simulink model "QD2_IMU_2021a"  (R2021a)
settings: Solver=ode2  StartTime=0.0  StopTime=inf  FixedStep=1/1000  RelTol=1e-3  EnableMultiTasking=on
undefined symbols (not defined in the file): HIL
libraries: quarc_library x7, simulink x2
settings Model: DataTypeOverride=Double  MinMaxOverflowLogging=ForceOff  SimulationMode=external  ExtModeTrigElement=1  ExtModeTrigDuration=10000  ExtModeTrigLevel=0.400000  Creator=dmadill  LastModifiedBy=lgonzalez
settings SolverCC: AlgebraicLoopSolver=TrustRegion  PositivePriorityOrder=on
settings DataIOCC: ReturnWorkspaceOutputs=off
settings DebuggingCC: SFMachineParentedDataDiag=warning  ArithmeticOperatorsInVariantConditions=warning
settings HardwareCC: ProdBitPerLong=64  ProdLargestAtomicInteger=LongLong  ProdLargestAtomicFloat=Double  ProdLongLongMode=on  ProdHWDeviceType=ARM Compatible->ARM 64-bit (LP64)
settings SFSimCC: SimUseLocalCustomCode=off  CustomCodeUndefinedFunction=UseInterfaceOnly
settings RTWCC: Description=QUARC Linux QDrone2 Target Using Toolchain  SystemTargetFile=quarc_linux_qdrone2.tlc  RTWUseLocalCustomCode=off  Toolchain=QUARC linux_qdrone2 | gmake (64-bit Windows)  BuildConfiguration=Faster Runs
settings CodeAppCC: StateflowObjectComments=on
settings STFCustomTargetCC: ConcurrentExecutionCompliant=on  SystemTargetFile=quarc_linux_qdrone2.tlc
settings GRTTargetCC: TargetLangStandard=C89/C90 (ANSI)  ParMdlRefBuildCompliant=off  CompOptLevelCompliant=off  CombineOutputUpdateFcns=off  MatFileLogging=off  CPPClassGenCompliant=off  GRTInterface=on  ExtMode=on  ExtModeMexFile=quarc_comm  ExtModeMexArgs='-w -d /tmp -uri %u','tcpip://192.168.2.d:17001'
settings ConfigComp: CovMetricSettings=dswe

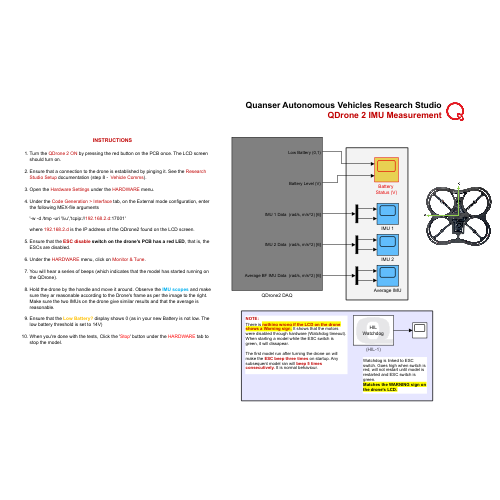
[thumbnail: Simulink's stored preview of the top-level diagram]
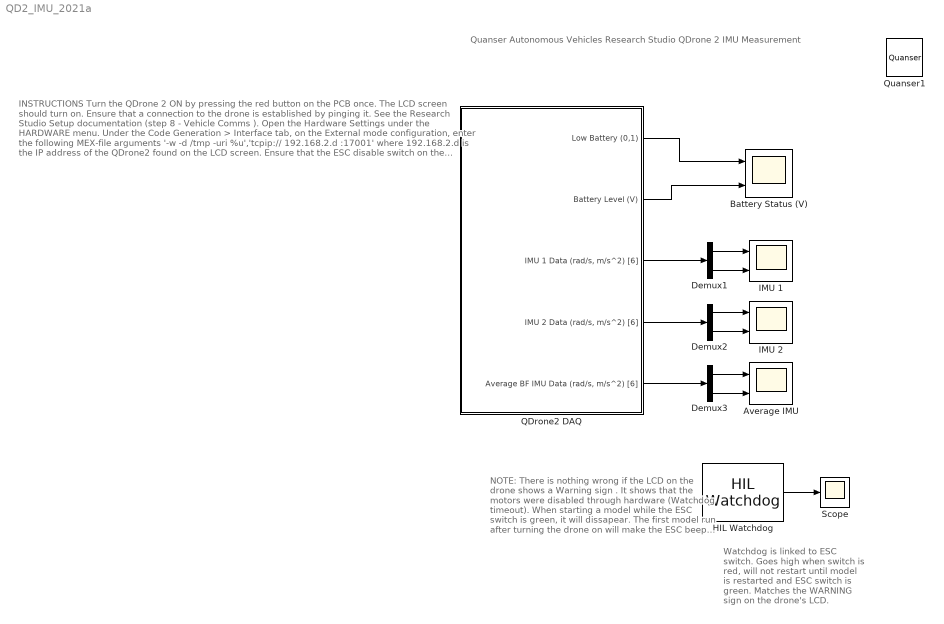
== system QD2_IMU_2021a ==
  note: Quanser Autonomous Vehicles Research Studio
      | QDrone 2 IMU Measurement
  note: Watchdog is linked to ESC switch. Goes high when switch is red, will not restart until model is restarted and ESC switch is green.
      | Matches the WARNING sign on the drone's LCD.
  note: NOTE:
      | There is nothing wrong if the LCD on the drone shows a Warning sign . It shows that the motors were disabled through hardware (Watchdog timeout). When starting a model while the ESC switch is green, it will dissapear.
      |
      | The first model run after turning the drone on will make the ESC beep three times on startup. Any subsequent model ran will beep 5 times consecutively. It is normal behaviour.
  note: INSTRUCTIONS
      |
      | Turn the QDrone 2 ON by pressing the red button on the PCB once. The LCD screen should turn on.
      |
      | Ensure that a connection to the drone is established by pinging it. See the Research Studio Setup documentation (step 8 - Vehicle Comms ).
      |
      | Open the Hardware Settings under the HARDWARE menu.
      |
      | Under the Code Generation > Interface tab, on the External mode configuration, enter the following MEX-file arguments
      |
      | '-w -d /tmp -uri %u','tcpip:// 192.168.2.d :17001'
      |
      | where 192.168.2.d is the IP address of the QDrone2 found on the LCD screen.
      |
      | Ensure that the ESC disable switch on the drone's PCB has a red LED , that is, the ESCs are disabled.
      |
      | Under the HARDWARE menu, click on Monitor & Tune .
      |
      | You will hear a series of beeps (which indicates that the model has started running on the QDrone).
      |
      | Hold the drone by the handle and move it around. Observe the IMU scopes and make sure they ar reasonable according to the Drone's frame as per the image to the right. Make sure the two IMUs on the drone give similar results and that the average is reasonable.
      |
      | Ensure that the Low Battery? display shows 0 (as in your new Battery is not low. The low battery threshold is set to 14V)
      |
      | When you're done with the tests, Click the ' Stop ' button under the HARDWARE tab to stop the model.
  Average IMU : Scope  NumInputPorts=2
  Battery Status (V) : Scope  NumInputPorts=2
  Demux1 : Demux  Outputs=2
  Demux2 : Demux  Outputs=2
  Demux3 : Demux  Outputs=2
  HIL Watchdog : quarc_library/Data Acquisition/Generic/Watchdog/HIL Watchdog  object_name=HIL-1  timeout=0.1  sample_time=qc_get_step_size  active=off
      settings: AttributesFormatString=(%<object_name>)  SourceProductName=QUARC Targets
  IMU 1 : Scope  NumInputPorts=2
  IMU 2 : Scope  NumInputPorts=2
  QDrone2 DAQ : Subsystem
  Quanser1 : quarc_library/Logos/Quanser
  Scope : Scope
  wires:
  QDrone2 DAQ/1(Low Battery (0,1)) -> Battery Status (V)/1
  QDrone2 DAQ/2(Battery Level (V)) -> Battery Status (V)/2
  HIL Watchdog/1 -> Scope/1
  QDrone2 DAQ/3("IMU 1 Data (rad/s, m/s^2) [6]") -> Demux1/1
  QDrone2 DAQ/4("IMU 2 Data (rad/s, m/s^2) [6]") -> Demux2/1
  Demux1/1 -> IMU 1/1
  Demux1/2 -> IMU 1/2
  Demux2/1 -> IMU 2/1
  Demux2/2 -> IMU 2/2
  Demux3/1 -> Average IMU/1
  Demux3/2 -> Average IMU/2
  QDrone2 DAQ/5("Average BF IMU Data (rad/s, m/s^2) [6]") -> Demux3/1

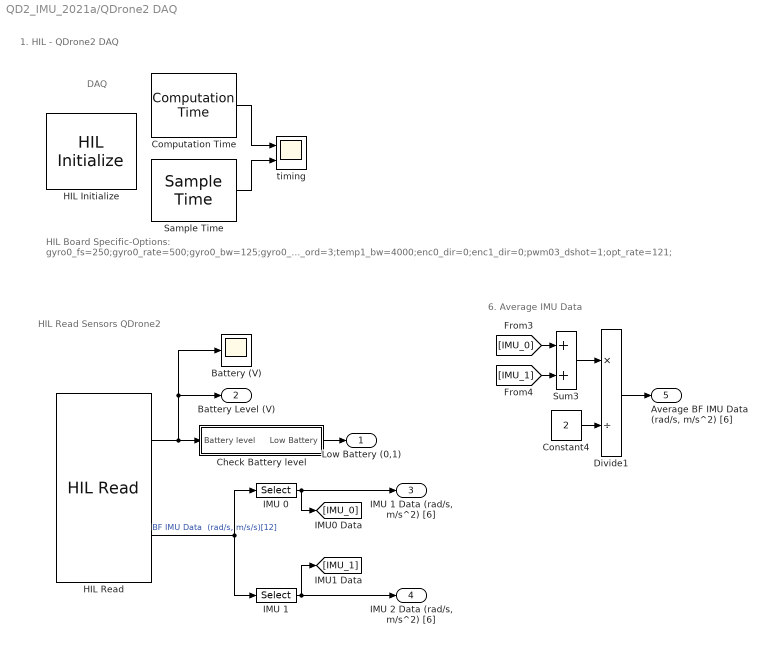
== system QD2_IMU_2021a/QDrone2 DAQ ==
  note: 1. HIL - QDrone2 DAQ
  note: DAQ
  note: HIL Read Sensors QDrone2
  note: 6. Average IMU Data
  note: HIL Board Specific-Options:
      | gyro0_fs=250;gyro0_rate=500;gyro0_bw=125;gyro0_ord=3;accel0_fs=16;accel0_rate=1000;accel0_bw=400;accel0_ord=3;temp0_bw=4000;gyro1_fs=250;gyro1_rate=500;gyro1_bw=125;gyro1_ord=3;accel1_fs=16;accel1_rate=1000;accel1_bw=400;accel1_ord=3;temp1_bw=4000;enc0_dir=0;enc1_dir=0;pwm03_dshot=1;opt_rate=121;
  Battery (V) : Scope
  Check Battery level : Subsystem
  Computation Time : quarc_library/Sources/Time/Computation Time  sample_time=qc_get_step_size  use_model=on  use_cpu_time=off
  Constant4 : Constant  Value=2
  Divide1 : Product  Inputs=*/
  HIL Initialize : quarc_library/Data Acquisition/Generic/Configuration/HIL Initialize  object_name=HIL-1  board_type=qdrone2  board_number=0  board_options=gyro0_fs=250;gyro0_rate=500;gyro0_bw=125;gyro0_ord=3;accel0_fs=16;accel0_rate=1000;accel0_bw=400;accel0_ord=3;temp0_bw=4000;gyro1_fs=250;gyro1_rate=500;gyro1_bw=125;gyro1_ord=3;accel1_fs=16;accel1_rate=1000;accel1_bw=400;accel1_ord=3;temp1_bw=4000;enc0_dir=0;enc1_dir=0;pwm03_dshot=1;opt_rate=121;  exclusive=off  active=on  hardware_clocks=[]  clock_modes=[]  initial_clock_frequencies=[]  set_clock_params_at_start=off  set_clock_params_at_switch_in=off  set_clock_frequencies_at_start=off  set_clock_frequencies_at_switch_in=off  analog_input_channels=[0:3]  analog_input_configurations=[]  analog_input_maximums=[3.3]  analog_input_minimums=[0]  set_analog_input_params_at_start=off  set_analog_input_params_at_switch_in=off  analog_output_channels=[]  analog_output_maximums=[]  analog_output_minimums=[]  initial_analog_outputs=[]  final_analog_outputs=[]  watchdog_analog_outputs=[]  set_analog_output_params_at_start=off  set_analog_output_params_at_switch_in=off  set_analog_outputs_at_start=off  set_analog_outputs_at_switch_in=off  set_analog_outputs_at_terminate=off  set_analog_outputs_at_switch_out=off  set_analog_outputs_on_watchdog=off  digital_input_channels=[0:5]  digital_output_channels=[6:11]  digital_output_configuration=[]  initial_digital_outputs=[0]  final_digital_outputs=[0]  watchdog_digital_outputs=[0 0 0 0 0 0]  set_digital_output_params_at_start=off  set_digital_output_params_at_switch_in=off  set_digital_outputs_at_start=on  set_digital_outputs_at_switch_in=off  set_digital_outputs_at_terminate=on  set_digital_outputs_at_switch_out=off  set_digital_outputs_on_watchdog=off  encoder_channels=[0:1]  quadrature=[4]  encoder_filter_frequency=100e6/1  initial_encoder_counts=[0]  set_encoder_params_at_start=on  set_encoder_params_at_switch_in=off  set_encoder_counts_at_start=on  set_encoder_counts_at_switch_in=off  pwm_channels=[0:5]  pwm_modes=[6 6 6 6 0 0]  pwm_frequency=1.2e6  pwm_configuration=[0]  pwm_alignment=[0]  pwm_polarity=[1]  pwm_leading_deadband=[]  pwm_trailing_deadband=[]  initial_pwm_outputs=[0]  final_pwm_outputs=[0]  watchdog_pwm_outputs=[0]  set_pwm_params_at_start=on  set_pwm_params_at_switch_in=off  set_pwm_outputs_at_start=on  set_pwm_outputs_at_switch_in=off  set_pwm_outputs_at_terminate=on  set_pwm_outputs_at_switch_out=off  set_pwm_outputs_on_watchdog=on  other_output_channels=[]  initial_other_outputs=[]  final_other_outputs=[]  watchdog_other_outputs=[]  set_other_outputs_at_start=on  set_other_outputs_at_switch_in=off  set_other_outputs_at_terminate=on  set_other_outputs_at_switch_out=off  set_other_outputs_on_watchdog=off
  HIL Read : quarc_library/Data Acquisition/Generic/Immediate I//O/HIL Read  object_name=HIL-1  analog_channels=[3]  encoder_channels=[]  digital_channels=[]  other_channels=[3000:3002 4000:4002 3003:3005 4003:4005]  sample_time=qc_get_step_size  active=on  vector_output=on  data_type_mode=Inherit via back propagation  encoder_data_type=double  digital_data_type=boolean
  IMU 0 : Selector  InputPortWidth=12  IndexOptions=Index vector (dialog)  Indices=[1:6]  OutputSizes=1
  IMU 1 : Selector  InputPortWidth=12  IndexOptions=Index vector (dialog)  Indices=[7:12]  OutputSizes=1
  Sample Time : quarc_library/Sources/Time/Sample Time  Priority=-99  sample_time=qc_get_step_size
  Sum3 : Sum
  timing : Scope  NumInputPorts=2
  Low Battery (0,1) : Outport
  Battery Level (V) : Outport  Port=2
  "IMU 1 Data (rad/s, m/s^2) [6]" : Outport  Port=3
  "IMU 2 Data (rad/s, m/s^2) [6]" : Outport  Port=4
  "Average BF IMU Data (rad/s, m/s^2) [6]" : Outport  Port=5
  wires:
  Check Battery level/1(Low Battery) -> Low Battery (0,1)/1
  IMU 1/1 -> [IMU_1], "IMU 2 Data (rad/s, m/s^2) [6]"/1
  IMU 0/1 -> "IMU 1 Data (rad/s, m/s^2) [6]"/1, [IMU_0]
  HIL Read/1 -> Battery (V)/1, Battery Level (V)/1, Check Battery level/1(Battery level)
  HIL Read/2 -> IMU 0/1, IMU 1/1  "BF IMU Data  (rad/s, m/s/s)[12]"
  [IMU_0] -> Sum3/1
  Sum3/1 -> Divide1/1
  Divide1/1 -> "Average BF IMU Data (rad/s, m/s^2) [6]"/1
  Constant4/1 -> Divide1/2
  [IMU_1] -> Sum3/2
  Sample Time/1 -> timing/2
  Computation Time/1 -> timing/1

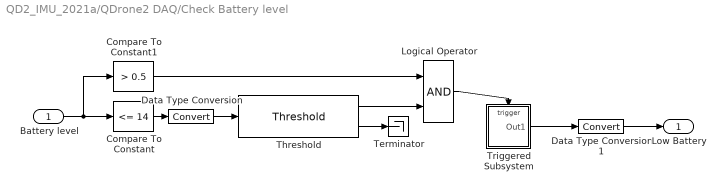
== system QD2_IMU_2021a/QDrone2 DAQ/Check Battery level ==
  Battery level : Inport
  Compare To Constant : simulink/Logic and Bit Operations/Compare To Constant  relop=<=  const=14  OutDataTypeStr=boolean
  Compare To Constant1 : simulink/Logic and Bit Operations/Compare To Constant  relop=>  const=0.5  OutDataTypeStr=boolean
  Data Type Conversion : DataTypeConversion
  Data Type Conversion1 : DataTypeConversion
  Logical Operator : Logic  AllPortsSameDT=off  OutDataTypeStr=boolean
  Terminator : Terminator
  Threshold : quarc_library/Discontinuities/Threshold  operator=>=  param_src=Specify via dialog  threshold=0.5  duration=0.3
      settings: SourceProductName=QUARC Targets
  Triggered Subsystem : Subsystem  TreatAsAtomicUnit=on
  Low Battery : Outport  VectorParamsAs1DForOutWhenUnconnected=off
  wires:
  Threshold/2 -> Terminator/1
  Battery level/1 -> Compare To Constant1/1, Compare To Constant/1
  Threshold/1 -> Logical Operator/2
  Logical Operator/1 -> Triggered Subsystem/Trigger
  Compare To Constant1/1 -> Logical Operator/1
  Compare To Constant/1 -> Data Type Conversion/1
  Data Type Conversion/1 -> Threshold/1
  Data Type Conversion1/1 -> Low Battery/1
  Triggered Subsystem/1(Out1) -> Data Type Conversion1/1

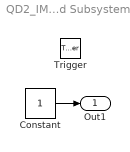
== system QD2_IMU_2021a/QDrone2 DAQ/Check Battery level/Triggered Subsystem ==
  Trigger : TriggerPort  VariantControl=(inherit)
  Constant : Constant
  Out1 : Outport  InitialOutput=[0]
  wires:
  Constant/1 -> Out1/1
